simulink model "exercise3"  (R2019b)
settings: Solver=VariableStepAuto  StartTime=0.0  StopTime=10.0  RelTol=1e-3
libraries: simulink x1
settings Model: Creator=hp  LastModifiedBy=hp

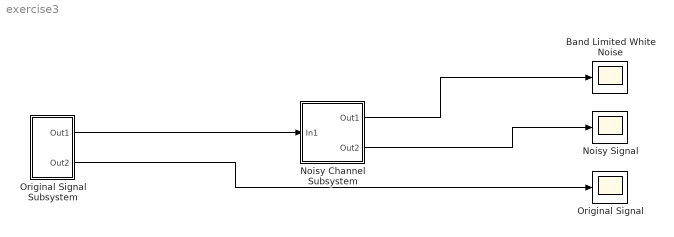
== system exercise3 ==
  "Band Limited White Noise " : Scope  NumInputPorts=3
  "Noisy Channel Subsystem " : Subsystem
  "Noisy Signal " : Scope  NumInputPorts=3
  "Original Signal " : Scope  NumInputPorts=3
  "Original Signal Subsystem " : Subsystem
  wires:
  "Original Signal Subsystem "/2(Out2) -> "Original Signal "/2
  "Original Signal Subsystem "/1(Out1) -> "Noisy Channel Subsystem "/1(In1)
  "Noisy Channel Subsystem "/1(Out1) -> "Band Limited White Noise "/2
  "Noisy Channel Subsystem "/2(Out2) -> "Noisy Signal "/2

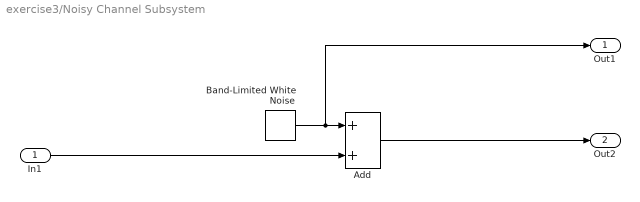
== system exercise3/Noisy Channel Subsystem  ==
  In1 : Inport
  Add : Sum
  Band-Limited White Noise : simulink/Sources/Band-Limited White Noise  Cov=[0.1]  Ts=0.1  seed=[23341]
  Out1 : Outport
  Out2 : Outport  Port=2
  wires:
  In1/1 -> Add/2
  Band-Limited White Noise/1 -> Out1/1, Add/1
  Add/1 -> Out2/1

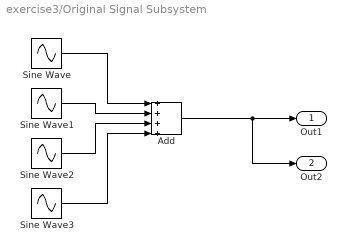
== system exercise3/Original Signal Subsystem  ==
  Add : Sum  Inputs=++++
  Sine Wave : Sin  Frequency=100  SampleTime=0
  Sine Wave1 : Sin  Frequency=9788  SampleTime=0
  Sine Wave2 : Sin  Frequency=3451  SampleTime=0
  Sine Wave3 : Sin  Frequency=2  SampleTime=0
  Out1 : Outport
  Out2 : Outport  Port=2
  wires:
  Sine Wave1/1 -> Add/2
  Sine Wave/1 -> Add/1
  Sine Wave3/1 -> Add/4
  Add/1 -> Out2/1, Out1/1
  Sine Wave2/1 -> Add/3
